simulink model "test_mdl"  (R2018a)
settings: Solver=VariableStepAuto  StartTime=0.0  StopTime=10.0  RelTol=1e-3
(part 8 of 8)

== system test_mdl/FD1_CAN_P702_GASD_MY21_DCV_V06/SOBDMC_HPCM_FD1/PreCond_Hev_Data2_FD1 ==
  BattTracClntFlw_Pc_Rq : Constant
  BattTrac_I_EstVsc : Constant
  DrvCondTpRrDefrs_B_Rq : Constant
  HtrnAin_UHi_Actl : Constant
  HtrnHvilOpen_B_Actl : Constant
  HtrnMil_D_Rq : Constant
  HtrnOvrTeLamp_B_Dsply : Constant
  HtrnSrvcRqd_B_Dsply : Constant
  PreCondActv_B_Actl : Constant
  PtWakeupDeltaT_T_Rq : Constant
  bus_creator : BusCreator  Inputs=10
  port : Outport
  wires:
  bus_creator/1 -> port/1  "PreCond_Hev_Data2_FD1"
  BattTracClntFlw_Pc_Rq/1 -> bus_creator/1  "BattTracClntFlw_Pc_Rq"
  BattTrac_I_EstVsc/1 -> bus_creator/2  "BattTrac_I_EstVsc"
  DrvCondTpRrDefrs_B_Rq/1 -> bus_creator/3  "DrvCondTpRrDefrs_B_Rq"
  HtrnAin_UHi_Actl/1 -> bus_creator/4  "HtrnAin_UHi_Actl"
  HtrnHvilOpen_B_Actl/1 -> bus_creator/5  "HtrnHvilOpen_B_Actl"
  HtrnMil_D_Rq/1 -> bus_creator/6  "HtrnMil_D_Rq"
  HtrnOvrTeLamp_B_Dsply/1 -> bus_creator/7  "HtrnOvrTeLamp_B_Dsply"
  HtrnSrvcRqd_B_Dsply/1 -> bus_creator/8  "HtrnSrvcRqd_B_Dsply"
  PreCondActv_B_Actl/1 -> bus_creator/9  "PreCondActv_B_Actl"
  PtWakeupDeltaT_T_Rq/1 -> bus_creator/10  "PtWakeupDeltaT_T_Rq"

== system test_mdl/FD1_CAN_P702_GASD_MY21_DCV_V06/SOBDMC_HPCM_FD1/SOBDMC_AutoSar_NetMgmt_FD1 ==
  SOBDMC_AutoSarNMControl : Constant
  SOBDMC_AutoSarNMNodeId : Constant
  SOBDMC_AutoSarNMReserved{1..4} (4 alike) : Constant
  SOBDMC_GWNMProxy : Constant
  SOBDMC_GWOnBoardTester : Constant
  bus_creator : BusCreator  Inputs=8
  port : Outport
  wires:
  bus_creator/1 -> port/1  "SOBDMC_AutoSar_NetMgmt_FD1"
  SOBDMC_AutoSarNMControl/1 -> bus_creator/1  "SOBDMC_AutoSarNMControl"
  SOBDMC_AutoSarNMNodeId/1 -> bus_creator/2  "SOBDMC_AutoSarNMNodeId"
  SOBDMC_AutoSarNMReserved1/1 -> bus_creator/3  "SOBDMC_AutoSarNMReserved1"
  SOBDMC_AutoSarNMReserved2/1 -> bus_creator/4  "SOBDMC_AutoSarNMReserved2"
  SOBDMC_AutoSarNMReserved3/1 -> bus_creator/5  "SOBDMC_AutoSarNMReserved3"
  SOBDMC_AutoSarNMReserved4/1 -> bus_creator/6  "SOBDMC_AutoSarNMReserved4"
  SOBDMC_GWNMProxy/1 -> bus_creator/7  "SOBDMC_GWNMProxy"
  SOBDMC_GWOnBoardTester/1 -> bus_creator/8  "SOBDMC_GWOnBoardTester"

== system test_mdl/FD1_CAN_P702_GASD_MY21_DCV_V06/SOBDMC_HPCM_FD1/SOBDMC_RapidData_Resp1_FD1 ==
  UUDTSOBDMCResponse1 : Constant
  bus_creator : BusCreator  Inputs=1
  port : Outport
  wires:
  bus_creator/1 -> port/1  "SOBDMC_RapidData_Resp1_FD1"
  UUDTSOBDMCResponse1/1 -> bus_creator/1  "UUDTSOBDMCResponse1"

== system test_mdl/FD1_CAN_P702_GASD_MY21_DCV_V06/SOBDMC_HPCM_FD1/SOBDMC_RapidData_Resp2_FD1 ==
  UUDTSOBDMCResponse2 : Constant
  bus_creator : BusCreator  Inputs=1
  port : Outport
  wires:
  bus_creator/1 -> port/1  "SOBDMC_RapidData_Resp2_FD1"
  UUDTSOBDMCResponse2/1 -> bus_creator/1  "UUDTSOBDMCResponse2"

== system test_mdl/FD1_CAN_P702_GASD_MY21_DCV_V06/SOBDMC_HPCM_FD1/SOBDMC_RapidData_Resp3_FD1 ==
  UUDTSOBDMCResponse3 : Constant
  bus_creator : BusCreator  Inputs=1
  port : Outport
  wires:
  bus_creator/1 -> port/1  "SOBDMC_RapidData_Resp3_FD1"
  UUDTSOBDMCResponse3/1 -> bus_creator/1  "UUDTSOBDMCResponse3"

== system test_mdl/FD1_CAN_P702_GASD_MY21_DCV_V06/SOBDMC_HPCM_FD1/SOBDMC_RapidData_Resp4_FD1 ==
  UUDTSOBDMCResponse4 : Constant
  bus_creator : BusCreator  Inputs=1
  port : Outport
  wires:
  bus_creator/1 -> port/1  "SOBDMC_RapidData_Resp4_FD1"
  UUDTSOBDMCResponse4/1 -> bus_creator/1  "UUDTSOBDMCResponse4"

== system test_mdl/FD1_CAN_P702_GASD_MY21_DCV_V06/SOBDMC_HPCM_FD1/Saved_Charge_Location_FD1 ==
  ChrgLocId_D_Sav : Constant
  ChrgLocLattDeg_An_Sav : Constant
  ChrgLocLattFrct_An_Sav : Constant
  ChrgLocLattPostv_B_Sav : Constant
  ChrgLocLongDeg_An_Sav : Constant
  ChrgLocLongFrct_An_Sav : Constant
  ChrgLocLongPostv_B_Sav : Constant
  ChrgLocSaved_B_Dsply : Constant
  ChrgNowCurnt_B_Dsply : Constant
  bus_creator : BusCreator  Inputs=9
  port : Outport
  wires:
  bus_creator/1 -> port/1  "Saved_Charge_Location_FD1"
  ChrgLocId_D_Sav/1 -> bus_creator/1  "ChrgLocId_D_Sav"
  ChrgLocLattDeg_An_Sav/1 -> bus_creator/2  "ChrgLocLattDeg_An_Sav"
  ChrgLocLattFrct_An_Sav/1 -> bus_creator/3  "ChrgLocLattFrct_An_Sav"
  ChrgLocLattPostv_B_Sav/1 -> bus_creator/4  "ChrgLocLattPostv_B_Sav"
  ChrgLocLongDeg_An_Sav/1 -> bus_creator/5  "ChrgLocLongDeg_An_Sav"
  ChrgLocLongFrct_An_Sav/1 -> bus_creator/6  "ChrgLocLongFrct_An_Sav"
  ChrgLocLongPostv_B_Sav/1 -> bus_creator/7  "ChrgLocLongPostv_B_Sav"
  ChrgLocSaved_B_Dsply/1 -> bus_creator/8  "ChrgLocSaved_B_Dsply"
  ChrgNowCurnt_B_Dsply/1 -> bus_creator/9  "ChrgNowCurnt_B_Dsply"

== system test_mdl/FD1_CAN_P702_GASD_MY21_DCV_V06/SOBDMC_HPCM_FD1/TesterPhysicalResSOBDMCFD1 ==
  TesterPhysicalResSOBDMC : Constant
  bus_creator : BusCreator  Inputs=1
  port : Outport
  wires:
  bus_creator/1 -> port/1  "TesterPhysicalResSOBDMCFD1"
  TesterPhysicalResSOBDMC/1 -> bus_creator/1  "TesterPhysicalResSOBDMC"

== system test_mdl/FD1_CAN_P702_GASD_MY21_DCV_V06/SOBDMC_HPCM_FD1/Unsaved_Charge_LocationFD1 ==
  ChrgLocId_D_Uns : Constant
  ChrgLocLattDeg_An_Uns : Constant
  ChrgLocLattFrct_An_Uns : Constant
  ChrgLocLattPostv_B_Uns : Constant
  ChrgLocLongDeg_An_Uns : Constant
  ChrgLocLongFrct_An_Uns : Constant
  ChrgLocLongPostv_B_Uns : Constant
  bus_creator : BusCreator  Inputs=7
  port : Outport
  wires:
  bus_creator/1 -> port/1  "Unsaved_Charge_LocationFD1"
  ChrgLocId_D_Uns/1 -> bus_creator/1  "ChrgLocId_D_Uns"
  ChrgLocLattDeg_An_Uns/1 -> bus_creator/2  "ChrgLocLattDeg_An_Uns"
  ChrgLocLattFrct_An_Uns/1 -> bus_creator/3  "ChrgLocLattFrct_An_Uns"
  ChrgLocLattPostv_B_Uns/1 -> bus_creator/4  "ChrgLocLattPostv_B_Uns"
  ChrgLocLongDeg_An_Uns/1 -> bus_creator/5  "ChrgLocLongDeg_An_Uns"
  ChrgLocLongFrct_An_Uns/1 -> bus_creator/6  "ChrgLocLongFrct_An_Uns"
  ChrgLocLongPostv_B_Uns/1 -> bus_creator/7  "ChrgLocLongPostv_B_Uns"

== system test_mdl/FD1_CAN_P702_GASD_MY21_DCV_V06/TCCM/AWD_Torque_Data ==
  PrplWhlTotTqRqMxAwd_No_Cnt : Constant
  PrplWhlTotTqRqMxAwd_No_Cs : Constant
  PrplWhlTot_Tq_RqMxAwd : Constant
  bus_creator : BusCreator  Inputs=3
  port : Outport
  wires:
  bus_creator/1 -> port/1  "AWD_Torque_Data"
  PrplWhlTotTqRqMxAwd_No_Cnt/1 -> bus_creator/1  "PrplWhlTotTqRqMxAwd_No_Cnt"
  PrplWhlTotTqRqMxAwd_No_Cs/1 -> bus_creator/2  "PrplWhlTotTqRqMxAwd_No_Cs"
  PrplWhlTot_Tq_RqMxAwd/1 -> bus_creator/3  "PrplWhlTot_Tq_RqMxAwd"

== system test_mdl/FD1_CAN_P702_GASD_MY21_DCV_V06/TCCM/Driveline_Data_1 ==
  Awd2wdLamp_D_RqDsply : Constant
  AwdAutoLamp_D_RqDsply : Constant
  AwdHiLamp_D_RqDsply : Constant
  AwdLck_D_Stat : Constant
  AwdLck_Tq_Rq : Constant
  AwdLoLamp_D_RqDsply : Constant
  AwdOffRoadMode_D_Stats : Constant
  AwdRnge_D_Actl : Constant
  AwdSrvcRqd_B_Rq : Constant
  AwdStat_D_RqDsply : Constant
  AwdSys_D_Stat : Constant
  NtrlTowAvail_B_Stat : Constant
  TrnAout_Tq_RqMx : Constant
  bus_creator : BusCreator  Inputs=13
  port : Outport
  wires:
  bus_creator/1 -> port/1  "Driveline_Data_1"
  Awd2wdLamp_D_RqDsply/1 -> bus_creator/1  "Awd2wdLamp_D_RqDsply"
  AwdAutoLamp_D_RqDsply/1 -> bus_creator/2  "AwdAutoLamp_D_RqDsply"
  AwdHiLamp_D_RqDsply/1 -> bus_creator/3  "AwdHiLamp_D_RqDsply"
  AwdLck_D_Stat/1 -> bus_creator/4  "AwdLck_D_Stat"
  AwdLck_Tq_Rq/1 -> bus_creator/5  "AwdLck_Tq_Rq"
  AwdLoLamp_D_RqDsply/1 -> bus_creator/6  "AwdLoLamp_D_RqDsply"
  AwdOffRoadMode_D_Stats/1 -> bus_creator/7  "AwdOffRoadMode_D_Stats"
  AwdRnge_D_Actl/1 -> bus_creator/8  "AwdRnge_D_Actl"
  AwdSrvcRqd_B_Rq/1 -> bus_creator/9  "AwdSrvcRqd_B_Rq"
  AwdStat_D_RqDsply/1 -> bus_creator/10  "AwdStat_D_RqDsply"
  AwdSys_D_Stat/1 -> bus_creator/11  "AwdSys_D_Stat"
  NtrlTowAvail_B_Stat/1 -> bus_creator/12  "NtrlTowAvail_B_Stat"
  TrnAout_Tq_RqMx/1 -> bus_creator/13  "TrnAout_Tq_RqMx"

== system test_mdl/FD1_CAN_P702_GASD_MY21_DCV_V06/TCCM/Driveline_Data_2 ==
  LsdSrvcRqd_B_Rq : Constant
  RearDiffFalt_D_Stat : Constant
  RearDiffLckLamp_D_Rq : Constant
  RearDiffLckMsg_D_Rq : Constant
  RearDiffLck_Tq_Actl : Constant
  SelDrvMdeAwd2_D_Stat : Constant
  bus_creator : BusCreator  Inputs=6
  port : Outport
  wires:
  bus_creator/1 -> port/1  "Driveline_Data_2"
  LsdSrvcRqd_B_Rq/1 -> bus_creator/1  "LsdSrvcRqd_B_Rq"
  RearDiffFalt_D_Stat/1 -> bus_creator/2  "RearDiffFalt_D_Stat"
  RearDiffLckLamp_D_Rq/1 -> bus_creator/3  "RearDiffLckLamp_D_Rq"
  RearDiffLckMsg_D_Rq/1 -> bus_creator/4  "RearDiffLckMsg_D_Rq"
  RearDiffLck_Tq_Actl/1 -> bus_creator/5  "RearDiffLck_Tq_Actl"
  SelDrvMdeAwd2_D_Stat/1 -> bus_creator/6  "SelDrvMdeAwd2_D_Stat"

== system test_mdl/FD1_CAN_P702_GASD_MY21_DCV_V06/TCCM/TCCM_AutoSar_NetwkMgmt ==
  TCCM_AutoSarNMControl : Constant
  TCCM_AutoSarNMNodeId : Constant
  TCCM_AutoSarNMReserved{1..4} (4 alike) : Constant
  TCCM_GWNMProxy : Constant
  TCCM_GWOnBoardTester : Constant
  bus_creator : BusCreator  Inputs=8
  port : Outport
  wires:
  bus_creator/1 -> port/1  "TCCM_AutoSar_NetwkMgmt"
  TCCM_AutoSarNMControl/1 -> bus_creator/1  "TCCM_AutoSarNMControl"
  TCCM_AutoSarNMNodeId/1 -> bus_creator/2  "TCCM_AutoSarNMNodeId"
  TCCM_AutoSarNMReserved1/1 -> bus_creator/3  "TCCM_AutoSarNMReserved1"
  TCCM_AutoSarNMReserved2/1 -> bus_creator/4  "TCCM_AutoSarNMReserved2"
  TCCM_AutoSarNMReserved3/1 -> bus_creator/5  "TCCM_AutoSarNMReserved3"
  TCCM_AutoSarNMReserved4/1 -> bus_creator/6  "TCCM_AutoSarNMReserved4"
  TCCM_GWNMProxy/1 -> bus_creator/7  "TCCM_GWNMProxy"
  TCCM_GWOnBoardTester/1 -> bus_creator/8  "TCCM_GWOnBoardTester"

== system test_mdl/FD1_CAN_P702_GASD_MY21_DCV_V06/TCCM/TesterPhysicalResTCCM ==
  TesterPhysicalResTCCM : Constant
  bus_creator : BusCreator  Inputs=1
  port : Outport
  wires:
  bus_creator/1 -> port/1  "TesterPhysicalResTCCM"
  TesterPhysicalResTCCM/1 -> bus_creator/1  "TesterPhysicalResTCCM"

== system test_mdl/FD1_CAN_P702_GASD_MY21_DCV_V06/TCM_DSL/EngineData_1 ==
  SeatWorkSrfc_B_Falt : Constant
  TrnIpcDsplyGear_D_Actl : Constant
  TrnIpcDsplyGear_D_Stat : Constant
  TrnIpcDsplyMde_D_Actl : Constant
  TrnIpcDsplyMde_D_Stat : Constant
  TrnIpcDsplyRng2_D_Actl : Constant
  TrnIpcDsplyRng_D_Stat : Constant
  bus_creator : BusCreator  Inputs=7
  port : Outport
  wires:
  bus_creator/1 -> port/1  "EngineData_1"
  SeatWorkSrfc_B_Falt/1 -> bus_creator/1  "SeatWorkSrfc_B_Falt"
  TrnIpcDsplyGear_D_Actl/1 -> bus_creator/2  "TrnIpcDsplyGear_D_Actl"
  TrnIpcDsplyGear_D_Stat/1 -> bus_creator/3  "TrnIpcDsplyGear_D_Stat"
  TrnIpcDsplyMde_D_Actl/1 -> bus_creator/4  "TrnIpcDsplyMde_D_Actl"
  TrnIpcDsplyMde_D_Stat/1 -> bus_creator/5  "TrnIpcDsplyMde_D_Stat"
  TrnIpcDsplyRng2_D_Actl/1 -> bus_creator/6  "TrnIpcDsplyRng2_D_Actl"
  TrnIpcDsplyRng_D_Stat/1 -> bus_creator/7  "TrnIpcDsplyRng_D_Stat"

== system test_mdl/FD1_CAN_P702_GASD_MY21_DCV_V06/TCM_DSL/Gear_Shift_by_Wire_3 ==
  GearSelLck_D_Rq : Constant
  PrkBrkActv_D_RqTrnGear : Constant
  TrnCmdCnt_B_Actl : Constant
  TrnCmdState_B_Actl : Constant
  TrnDtpCmd_D_Actl : Constant
  TrnGearCmd_No_Cnt : Constant
  TrnGearCmd_No_Cs : Constant
  TrnGearCmd_Pc_ActlPt : Constant
  TrnGearMsgTxt_D_Rq : Constant
  TrnGearNtmAllow_B_Stat : Constant
  TrnGear_D_RqPt : Constant
  TrnLvrV_D_Rq : Constant
  TrnNtrlTowCmd_D_Actl : Constant
  TrnSbwSysHlth_D_Actl : Constant
  TrnValidGear_D_Cnfm : Constant
  bus_creator : BusCreator  Inputs=15
  port : Outport
  wires:
  bus_creator/1 -> port/1  "Gear_Shift_by_Wire_3"
  GearSelLck_D_Rq/1 -> bus_creator/1  "GearSelLck_D_Rq"
  PrkBrkActv_D_RqTrnGear/1 -> bus_creator/2  "PrkBrkActv_D_RqTrnGear"
  TrnCmdCnt_B_Actl/1 -> bus_creator/3  "TrnCmdCnt_B_Actl"
  TrnCmdState_B_Actl/1 -> bus_creator/4  "TrnCmdState_B_Actl"
  TrnDtpCmd_D_Actl/1 -> bus_creator/5  "TrnDtpCmd_D_Actl"
  TrnGearCmd_No_Cnt/1 -> bus_creator/6  "TrnGearCmd_No_Cnt"
  TrnGearCmd_No_Cs/1 -> bus_creator/7  "TrnGearCmd_No_Cs"
  TrnGearCmd_Pc_ActlPt/1 -> bus_creator/8  "TrnGearCmd_Pc_ActlPt"
  TrnGearMsgTxt_D_Rq/1 -> bus_creator/9  "TrnGearMsgTxt_D_Rq"
  TrnGearNtmAllow_B_Stat/1 -> bus_creator/10  "TrnGearNtmAllow_B_Stat"
  TrnGear_D_RqPt/1 -> bus_creator/11  "TrnGear_D_RqPt"
  TrnLvrV_D_Rq/1 -> bus_creator/12  "TrnLvrV_D_Rq"
  TrnNtrlTowCmd_D_Actl/1 -> bus_creator/13  "TrnNtrlTowCmd_D_Actl"
  TrnSbwSysHlth_D_Actl/1 -> bus_creator/14  "TrnSbwSysHlth_D_Actl"
  TrnValidGear_D_Cnfm/1 -> bus_creator/15  "TrnValidGear_D_Cnfm"

== system test_mdl/FD1_CAN_P702_GASD_MY21_DCV_V06/TCM_DSL/PowertrainData_10 ==
  GearEngag_D_Actl : Constant
  GearLvr_D_ActlDrv : Constant
  GearPos_D_Actl : Constant
  GearPos_D_Trg : Constant
  GearPos_No_Cnt : Constant
  GearPos_No_Cs : Constant
  TrnIgnOffDly_T_Rq : Constant
  TrnPrkSys_D_Actl : Constant
  TrnRng_D_Rq : Constant
  bus_creator : BusCreator  Inputs=9
  port : Outport
  wires:
  bus_creator/1 -> port/1  "PowertrainData_10"
  GearEngag_D_Actl/1 -> bus_creator/1  "GearEngag_D_Actl"
  GearLvr_D_ActlDrv/1 -> bus_creator/2  "GearLvr_D_ActlDrv"
  GearPos_D_Actl/1 -> bus_creator/3  "GearPos_D_Actl"
  GearPos_D_Trg/1 -> bus_creator/4  "GearPos_D_Trg"
  GearPos_No_Cnt/1 -> bus_creator/5  "GearPos_No_Cnt"
  GearPos_No_Cs/1 -> bus_creator/6  "GearPos_No_Cs"
  TrnIgnOffDly_T_Rq/1 -> bus_creator/7  "TrnIgnOffDly_T_Rq"
  TrnPrkSys_D_Actl/1 -> bus_creator/8  "TrnPrkSys_D_Actl"
  TrnRng_D_Rq/1 -> bus_creator/9  "TrnRng_D_Rq"

== system test_mdl/FD1_CAN_P702_GASD_MY21_DCV_V06/TCM_DSL/TCM_AutoSar_NetworkMgt ==
  TCM_AutoSarNMControl : Constant
  TCM_AutoSarNMNodeId : Constant
  TCM_AutoSarNMReserved{1..4} (4 alike) : Constant
  TCM_GWNMProxy : Constant
  TCM_GWOnBoardTester : Constant
  bus_creator : BusCreator  Inputs=8
  port : Outport
  wires:
  bus_creator/1 -> port/1  "TCM_AutoSar_NetworkMgt"
  TCM_AutoSarNMControl/1 -> bus_creator/1  "TCM_AutoSarNMControl"
  TCM_AutoSarNMNodeId/1 -> bus_creator/2  "TCM_AutoSarNMNodeId"
  TCM_AutoSarNMReserved1/1 -> bus_creator/3  "TCM_AutoSarNMReserved1"
  TCM_AutoSarNMReserved2/1 -> bus_creator/4  "TCM_AutoSarNMReserved2"
  TCM_AutoSarNMReserved3/1 -> bus_creator/5  "TCM_AutoSarNMReserved3"
  TCM_AutoSarNMReserved4/1 -> bus_creator/6  "TCM_AutoSarNMReserved4"
  TCM_GWNMProxy/1 -> bus_creator/7  "TCM_GWNMProxy"
  TCM_GWOnBoardTester/1 -> bus_creator/8  "TCM_GWOnBoardTester"

== system test_mdl/FD1_CAN_P702_GASD_MY21_DCV_V06/TCM_DSL/TCM_Rapid_Data_Response_1 ==
  UUDTTCMResponse1 : Constant
  bus_creator : BusCreator  Inputs=1
  port : Outport
  wires:
  bus_creator/1 -> port/1  "TCM_Rapid_Data_Response_1"
  UUDTTCMResponse1/1 -> bus_creator/1  "UUDTTCMResponse1"

== system test_mdl/FD1_CAN_P702_GASD_MY21_DCV_V06/TCM_DSL/TCM_Rapid_Data_Response_2 ==
  UUDTTCMResponse2 : Constant
  bus_creator : BusCreator  Inputs=1
  port : Outport
  wires:
  bus_creator/1 -> port/1  "TCM_Rapid_Data_Response_2"
  UUDTTCMResponse2/1 -> bus_creator/1  "UUDTTCMResponse2"

== system test_mdl/FD1_CAN_P702_GASD_MY21_DCV_V06/TCM_DSL/TesterPhysicalResTCM ==
  TesterPhysicalResTCM : Constant
  bus_creator : BusCreator  Inputs=1
  port : Outport
  wires:
  bus_creator/1 -> port/1  "TesterPhysicalResTCM"
  TesterPhysicalResTCM/1 -> bus_creator/1  "TesterPhysicalResTCM"

== system test_mdl/FD1_CAN_P702_GASD_MY21_DCV_V06/TCM_DSL/TransData_3 ==
  TrnAout_W_ActlUnfilt : Constant
  bus_creator : BusCreator  Inputs=1
  port : Outport
  wires:
  bus_creator/1 -> port/1  "TransData_3"
  TrnAout_W_ActlUnfilt/1 -> bus_creator/1  "TrnAout_W_ActlUnfilt"

== system test_mdl/FD1_CAN_P702_GASD_MY21_DCV_V06/TCM_DSL/TransGearData ==
  GboxOil_Te_Actl : Constant
  GearLvrPos_D_Actl : Constant
  SelDrvMdeSwtch_D_Stat3 : Constant
  TrnShifActv_B_Actl : Constant
  TrnSrvcRqd_B_Rq : Constant
  bus_creator : BusCreator  Inputs=5
  port : Outport
  wires:
  bus_creator/1 -> port/1  "TransGearData"
  GboxOil_Te_Actl/1 -> bus_creator/1  "GboxOil_Te_Actl"
  GearLvrPos_D_Actl/1 -> bus_creator/2  "GearLvrPos_D_Actl"
  SelDrvMdeSwtch_D_Stat3/1 -> bus_creator/3  "SelDrvMdeSwtch_D_Stat3"
  TrnShifActv_B_Actl/1 -> bus_creator/4  "TrnShifActv_B_Actl"
  TrnSrvcRqd_B_Rq/1 -> bus_creator/5  "TrnSrvcRqd_B_Rq"

== system test_mdl/FD1_CAN_P702_GASD_MY21_DCV_V06/TCM_DSL/TransGearData_2 ==
  TrnMsgTxt2_D_Rq : Constant
  TrnMsgTxt_D_Rq : Constant
  bus_creator : BusCreator  Inputs=2
  port : Outport
  wires:
  bus_creator/1 -> port/1  "TransGearData_2"
  TrnMsgTxt2_D_Rq/1 -> bus_creator/1  "TrnMsgTxt2_D_Rq"
  TrnMsgTxt_D_Rq/1 -> bus_creator/2  "TrnMsgTxt_D_Rq"

== system test_mdl/FD1_CAN_P702_GASD_MY21_DCV_V06/TSTR/TesterFunctionalReq_FD1 ==
  TesterFunctionalReq : Constant
  bus_creator : BusCreator  Inputs=1
  port : Outport
  wires:
  bus_creator/1 -> port/1  "TesterFunctionalReq_FD1"
  TesterFunctionalReq/1 -> bus_creator/1  "TesterFunctionalReq"

== system test_mdl/FD1_CAN_P702_GASD_MY21_DCV_V06/TSTR/TesterPhysicalReqABS ==
  TesterPhysicalReqABS : Constant
  bus_creator : BusCreator  Inputs=1
  port : Outport
  wires:
  bus_creator/1 -> port/1  "TesterPhysicalReqABS"
  TesterPhysicalReqABS/1 -> bus_creator/1  "TesterPhysicalReqABS"

== system test_mdl/FD1_CAN_P702_GASD_MY21_DCV_V06/TSTR/TesterPhysicalReqCCM ==
  TesterPhysicalReqCCM : Constant
  bus_creator : BusCreator  Inputs=1
  port : Outport
  wires:
  bus_creator/1 -> port/1  "TesterPhysicalReqCCM"
  TesterPhysicalReqCCM/1 -> bus_creator/1  "TesterPhysicalReqCCM"

== system test_mdl/FD1_CAN_P702_GASD_MY21_DCV_V06/TSTR/TesterPhysicalReqCMR_DSMC ==
  TesterPhysicalReqCMR_DSMC : Constant
  bus_creator : BusCreator  Inputs=1
  port : Outport
  wires:
  bus_creator/1 -> port/1  "TesterPhysicalReqCMR_DSMC"
  TesterPhysicalReqCMR_DSMC/1 -> bus_creator/1  "TesterPhysicalReqCMR_DSMC"

== system test_mdl/FD1_CAN_P702_GASD_MY21_DCV_V06/TSTR/TesterPhysicalReqGWM_FD1 ==
  TesterPhysicalReqGWM_F1 : Constant
  bus_creator : BusCreator  Inputs=1
  port : Outport
  wires:
  bus_creator/1 -> port/1  "TesterPhysicalReqGWM_FD1"
  TesterPhysicalReqGWM_F1/1 -> bus_creator/1  "TesterPhysicalReqGWM_F1"

== system test_mdl/FD1_CAN_P702_GASD_MY21_DCV_V06/TSTR/TesterPhysicalReqIPMA ==
  TesterPhysicalReqIPMA : Constant
  bus_creator : BusCreator  Inputs=1
  port : Outport
  wires:
  bus_creator/1 -> port/1  "TesterPhysicalReqIPMA"
  TesterPhysicalReqIPMA/1 -> bus_creator/1  "TesterPhysicalReqIPMA"

== system test_mdl/FD1_CAN_P702_GASD_MY21_DCV_V06/TSTR/TesterPhysicalReqPCM ==
  TesterPhysicalReqPCM : Constant
  bus_creator : BusCreator  Inputs=1
  port : Outport
  wires:
  bus_creator/1 -> port/1  "TesterPhysicalReqPCM"
  TesterPhysicalReqPCM/1 -> bus_creator/1  "TesterPhysicalReqPCM"

== system test_mdl/FD1_CAN_P702_GASD_MY21_DCV_V06/TSTR/TesterPhysicalReqPSCM ==
  TesterPhysicalReqPSCM : Constant
  bus_creator : BusCreator  Inputs=1
  port : Outport
  wires:
  bus_creator/1 -> port/1  "TesterPhysicalReqPSCM"
  TesterPhysicalReqPSCM/1 -> bus_creator/1  "TesterPhysicalReqPSCM"

== system test_mdl/FD1_CAN_P702_GASD_MY21_DCV_V06/TSTR/TesterPhysicalReqSOBDMC_FD ==
  TesterPhysicalReqSOBDMC : Constant
  bus_creator : BusCreator  Inputs=1
  port : Outport
  wires:
  bus_creator/1 -> port/1  "TesterPhysicalReqSOBDMC_FD"
  TesterPhysicalReqSOBDMC/1 -> bus_creator/1  "TesterPhysicalReqSOBDMC"

== system test_mdl/FD1_CAN_P702_GASD_MY21_DCV_V06/TSTR/TesterPhysicalReqSODCMC ==
  TesterPhysicalReqSODCMC : Constant
  bus_creator : BusCreator  Inputs=1
  port : Outport
  wires:
  bus_creator/1 -> port/1  "TesterPhysicalReqSODCMC"
  TesterPhysicalReqSODCMC/1 -> bus_creator/1  "TesterPhysicalReqSODCMC"

== system test_mdl/FD1_CAN_P702_GASD_MY21_DCV_V06/TSTR/TesterPhysicalReqSODCMD ==
  TesterPhysicalReqSODCMD : Constant
  bus_creator : BusCreator  Inputs=1
  port : Outport
  wires:
  bus_creator/1 -> port/1  "TesterPhysicalReqSODCMD"
  TesterPhysicalReqSODCMD/1 -> bus_creator/1  "TesterPhysicalReqSODCMD"

== system test_mdl/FD1_CAN_P702_GASD_MY21_DCV_V06/TSTR/TesterPhysicalReqSODL ==
  TesterPhysicalReqSODL : Constant
  bus_creator : BusCreator  Inputs=1
  port : Outport
  wires:
  bus_creator/1 -> port/1  "TesterPhysicalReqSODL"
  TesterPhysicalReqSODL/1 -> bus_creator/1  "TesterPhysicalReqSODL"

== system test_mdl/FD1_CAN_P702_GASD_MY21_DCV_V06/TSTR/TesterPhysicalReqSODR ==
  TesterPhysicalReqSODR : Constant
  bus_creator : BusCreator  Inputs=1
  port : Outport
  wires:
  bus_creator/1 -> port/1  "TesterPhysicalReqSODR"
  TesterPhysicalReqSODR/1 -> bus_creator/1  "TesterPhysicalReqSODR"

== system test_mdl/FD1_CAN_P702_GASD_MY21_DCV_V06/TSTR/TesterPhysicalReqTCCM ==
  TesterPhysicalReqTCCM : Constant
  bus_creator : BusCreator  Inputs=1
  port : Outport
  wires:
  bus_creator/1 -> port/1  "TesterPhysicalReqTCCM"
  TesterPhysicalReqTCCM/1 -> bus_creator/1  "TesterPhysicalReqTCCM"

== system test_mdl/FD1_CAN_P702_GASD_MY21_DCV_V06/TSTR/TesterPhysicalReqTCM ==
  TesterPhysicalReqTCM : Constant
  bus_creator : BusCreator  Inputs=1
  port : Outport
  wires:
  bus_creator/1 -> port/1  "TesterPhysicalReqTCM"
  TesterPhysicalReqTCM/1 -> bus_creator/1  "TesterPhysicalReqTCM"

== system test_mdl/FD1_CAN_P702_GASD_MY21_DCV_V06/VDM/Suspension_Data ==
  SuspClkSync_No_Rq : Constant
  SuspFrntRight_L_Actl : Constant
  SuspFrnt_L_Actl : Constant
  SuspFrnt_L_Prev : Constant
  SuspRearRight_L_Actl : Constant
  SuspRear_L_Actl : Constant
  SuspRear_L_Prev : Constant
  bus_creator : BusCreator  Inputs=7
  port : Outport
  wires:
  bus_creator/1 -> port/1  "Suspension_Data"
  SuspClkSync_No_Rq/1 -> bus_creator/1  "SuspClkSync_No_Rq"
  SuspFrntRight_L_Actl/1 -> bus_creator/2  "SuspFrntRight_L_Actl"
  SuspFrnt_L_Actl/1 -> bus_creator/3  "SuspFrnt_L_Actl"
  SuspFrnt_L_Prev/1 -> bus_creator/4  "SuspFrnt_L_Prev"
  SuspRearRight_L_Actl/1 -> bus_creator/5  "SuspRearRight_L_Actl"
  SuspRear_L_Actl/1 -> bus_creator/6  "SuspRear_L_Actl"
  SuspRear_L_Prev/1 -> bus_creator/7  "SuspRear_L_Prev"

== system test_mdl/FD1_CAN_P702_GASD_MY21_DCV_V06/VDM/TesterPhysicalResVDM ==
  TesterPhysicalResVDM : Constant
  bus_creator : BusCreator  Inputs=1
  port : Outport
  wires:
  bus_creator/1 -> port/1  "TesterPhysicalResVDM"
  TesterPhysicalResVDM/1 -> bus_creator/1  "TesterPhysicalResVDM"

== system test_mdl/FD1_CAN_P702_GASD_MY21_DCV_V06/VDM/VeyDynamics_Data ==
  AdptDrvMdeChassis_D_Rq : Constant
  AdptDrvMdePt_D_Rq : Constant
  CcdMsgTxt_D_RqDsply : Constant
  Ccd_B_Falt : Constant
  SelDrvMdeSusp_D_Stat : Constant
  bus_creator : BusCreator  Inputs=5
  port : Outport
  wires:
  bus_creator/1 -> port/1  "VeyDynamics_Data"
  AdptDrvMdeChassis_D_Rq/1 -> bus_creator/1  "AdptDrvMdeChassis_D_Rq"
  AdptDrvMdePt_D_Rq/1 -> bus_creator/2  "AdptDrvMdePt_D_Rq"
  CcdMsgTxt_D_RqDsply/1 -> bus_creator/3  "CcdMsgTxt_D_RqDsply"
  Ccd_B_Falt/1 -> bus_creator/4  "Ccd_B_Falt"
  SelDrvMdeSusp_D_Stat/1 -> bus_creator/5  "SelDrvMdeSusp_D_Stat"
